simulink model "sensorFusion_block"  (R2022b)
settings: Solver=ode8  StartTime=0.0  StopTime=10.0  FixedStep=dt  RelTol=1e-3
settings Model: Creator=lasto  LastModifiedBy=lasto

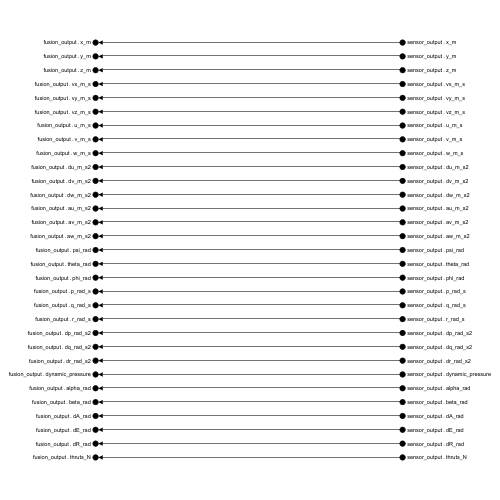
[thumbnail: Simulink's stored preview of the top-level diagram]
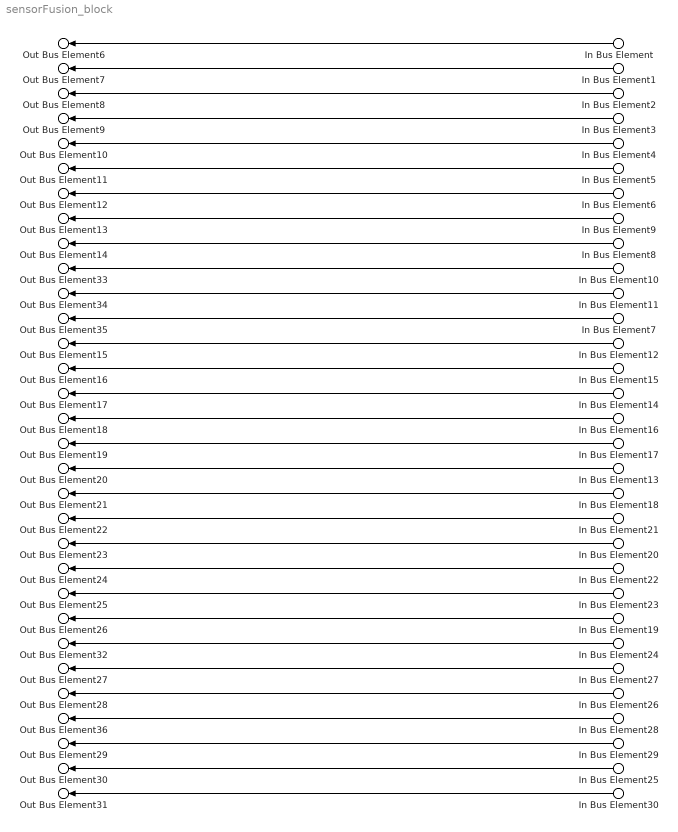
== system sensorFusion_block ==
  In Bus Element : Inport  PortName=sensor_output  Element=x_m
  In Bus Element5 : Inport  PortName=sensor_output  Element=vz_m_s
  In Bus Element2 : Inport  PortName=sensor_output  Element=z_m
  In Bus Element1 : Inport  PortName=sensor_output  Element=y_m
  In Bus Element3 : Inport  PortName=sensor_output  Element=vx_m_s
  In Bus Element4 : Inport  PortName=sensor_output  Element=vy_m_s
  In Bus Element6 : Inport  PortName=sensor_output  Element=u_m_s
  In Bus Element9 : Inport  PortName=sensor_output  Element=v_m_s
  In Bus Element8 : Inport  PortName=sensor_output  Element=w_m_s
  In Bus Element10 : Inport  PortName=sensor_output  Element=du_m_s2
  In Bus Element11 : Inport  PortName=sensor_output  Element=dv_m_s2
  In Bus Element7 : Inport  PortName=sensor_output  Element=dw_m_s2
  In Bus Element12 : Inport  PortName=sensor_output  Element=au_m_s2
  In Bus Element15 : Inport  PortName=sensor_output  Element=av_m_s2
  In Bus Element14 : Inport  PortName=sensor_output  Element=aw_m_s2
  In Bus Element16 : Inport  PortName=sensor_output  Element=psi_rad
  In Bus Element17 : Inport  PortName=sensor_output  Element=theta_rad
  In Bus Element13 : Inport  PortName=sensor_output  Element=phi_rad
  In Bus Element18 : Inport  PortName=sensor_output  Element=p_rad_s
  In Bus Element21 : Inport  PortName=sensor_output  Element=q_rad_s
  In Bus Element20 : Inport  PortName=sensor_output  Element=r_rad_s
  In Bus Element22 : Inport  PortName=sensor_output  Element=dp_rad_s2
  In Bus Element23 : Inport  PortName=sensor_output  Element=dq_rad_s2
  In Bus Element19 : Inport  PortName=sensor_output  Element=dr_rad_s2
  In Bus Element24 : Inport  PortName=sensor_output  Element=dynamic_pressure
  In Bus Element27 : Inport  PortName=sensor_output  Element=alpha_rad
  In Bus Element26 : Inport  PortName=sensor_output  Element=beta_rad
  In Bus Element28 : Inport  PortName=sensor_output  Element=dA_rad
  In Bus Element29 : Inport  PortName=sensor_output  Element=dE_rad
  In Bus Element25 : Inport  PortName=sensor_output  Element=dR_rad
  In Bus Element30 : Inport  PortName=sensor_output  Element=thruts_N
  Out Bus Element6 : Outport  PortName=fusion_output  Element=x_m
  Out Bus Element7 : Outport  PortName=fusion_output  Element=y_m
  Out Bus Element8 : Outport  PortName=fusion_output  Element=z_m
  Out Bus Element9 : Outport  PortName=fusion_output  Element=vx_m_s
  Out Bus Element10 : Outport  PortName=fusion_output  Element=vy_m_s
  Out Bus Element11 : Outport  PortName=fusion_output  Element=vz_m_s
  Out Bus Element12 : Outport  PortName=fusion_output  Element=u_m_s
  Out Bus Element13 : Outport  PortName=fusion_output  Element=v_m_s
  Out Bus Element14 : Outport  PortName=fusion_output  Element=w_m_s
  Out Bus Element15 : Outport  PortName=fusion_output  Element=au_m_s2
  Out Bus Element16 : Outport  PortName=fusion_output  Element=av_m_s2
  Out Bus Element17 : Outport  PortName=fusion_output  Element=aw_m_s2
  Out Bus Element18 : Outport  PortName=fusion_output  Element=psi_rad
  Out Bus Element19 : Outport  PortName=fusion_output  Element=theta_rad
  Out Bus Element20 : Outport  PortName=fusion_output  Element=phi_rad
  Out Bus Element21 : Outport  PortName=fusion_output  Element=p_rad_s
  Out Bus Element22 : Outport  PortName=fusion_output  Element=q_rad_s
  Out Bus Element23 : Outport  PortName=fusion_output  Element=r_rad_s
  Out Bus Element24 : Outport  PortName=fusion_output  Element=dp_rad_s2
  Out Bus Element25 : Outport  PortName=fusion_output  Element=dq_rad_s2
  Out Bus Element26 : Outport  PortName=fusion_output  Element=dr_rad_s2
  Out Bus Element27 : Outport  PortName=fusion_output  Element=alpha_rad
  Out Bus Element28 : Outport  PortName=fusion_output  Element=beta_rad
  Out Bus Element29 : Outport  PortName=fusion_output  Element=dE_rad
  Out Bus Element30 : Outport  PortName=fusion_output  Element=dR_rad
  Out Bus Element31 : Outport  PortName=fusion_output  Element=thruts_N
  Out Bus Element32 : Outport  PortName=fusion_output  Element=dynamic_pressure
  Out Bus Element33 : Outport  PortName=fusion_output  Element=du_m_s2
  Out Bus Element34 : Outport  PortName=fusion_output  Element=dv_m_s2
  Out Bus Element35 : Outport  PortName=fusion_output  Element=dw_m_s2
  Out Bus Element36 : Outport  PortName=fusion_output  Element=dA_rad
  wires:
  In Bus Element24/1 -> Out Bus Element32/1
  In Bus Element21/1 -> Out Bus Element22/1
  In Bus Element6/1 -> Out Bus Element12/1
  In Bus Element16/1 -> Out Bus Element18/1
  In Bus Element9/1 -> Out Bus Element13/1
  In Bus Element1/1 -> Out Bus Element7/1
  In Bus Element23/1 -> Out Bus Element25/1
  In Bus Element28/1 -> Out Bus Element36/1
  In Bus Element27/1 -> Out Bus Element27/1
  In Bus Element12/1 -> Out Bus Element15/1
  In Bus Element18/1 -> Out Bus Element21/1
  In Bus Element25/1 -> Out Bus Element30/1
  In Bus Element/1 -> Out Bus Element6/1
  In Bus Element22/1 -> Out Bus Element24/1
  In Bus Element11/1 -> Out Bus Element34/1
  In Bus Element4/1 -> Out Bus Element10/1
  In Bus Element15/1 -> Out Bus Element16/1
  In Bus Element3/1 -> Out Bus Element9/1
  In Bus Element17/1 -> Out Bus Element19/1
  In Bus Element20/1 -> Out Bus Element23/1
  In Bus Element14/1 -> Out Bus Element17/1
  In Bus Element30/1 -> Out Bus Element31/1
  In Bus Element19/1 -> Out Bus Element26/1
  In Bus Element29/1 -> Out Bus Element29/1
  In Bus Element2/1 -> Out Bus Element8/1
  In Bus Element10/1 -> Out Bus Element33/1
  In Bus Element26/1 -> Out Bus Element28/1
  In Bus Element8/1 -> Out Bus Element14/1
  In Bus Element7/1 -> Out Bus Element35/1
  In Bus Element5/1 -> Out Bus Element11/1
  In Bus Element13/1 -> Out Bus Element20/1
